simulink library "commphrec2"  (Simulink 6.0)
settings: Solver=ode45  SolverMode=SingleTasking  StartTime=0.0  StopTime=10.0  RelTol=1e-3
undefined symbols (not defined in the file or in its folder): D
libraries: commblksprivate x6, dspbuff3 x2, dspsigattribs x2, dspmathops x2, dspmtrx3 x2, simulink_extras x2
settings Model: Creator=akansal  LastModifiedBy=jli  ProdHWDeviceType=Specified
settings DataIOCC: SignalLoggingName=logsOut
settings OptimizationCC: BooleanDataType=off
settings DebuggingCC: CheckExecutionContextPreStartOutputMsg=on  CheckExecutionContextRuntimeOutputMsg=on  SolverPrmCheckMsg=none
settings HardwareCC: ProdHWDeviceType=Specified
settings ModelReferenceCC: UpdateModelReferenceTargets=IfOutOfDate
settings GRTTargetCC: LifeSpan=inf
settings SFSimCC: SFSimApplyToAllLibs=on  SFSimBuildMode=Incremental

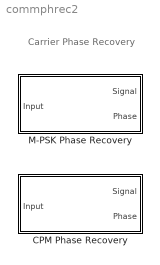
== system commphrec2 ==
  note: Carrier Phase Recovery
  CPM Phase Recovery : Subsystem  EnableExecutionContextPropagation=on  mask(CPM Phase Recovery){P=2, intPeriod=100}
      mask prompts: intPeriod "Observation interval (symbols):"
      mask help:
      | Recover the carrier phase using the 2P-Power method.  This non-data-aided, clock-aided feedforward method is suitable for full response CPM signals.
      |
      | The parameter P is the denominator of the modulation index (h=K/P) when expressed as a proper fraction. The observation interval parameter must be an integer multiple of the input signal vector length.
      mask init:
      | if ( ~isscalar(P) || (floor(P)~=P) )
      | 	error('P parameter must be an integer scalar.');
      | end
      | 
      | if ( ~isscalar(intPeriod) || (floor(intPeriod)~=intPeriod) )
      | 	error('The observation interval parameter must be an integer scalar.');
      | end
      mask Help: helpview(commbhelp);
      mask Display:
      | disp('CPM\nPhase Recovery');
      | port_label('output',1,'Sig');
      | port_label('output',2,'Ph');
  M-PSK Phase Recovery : Subsystem  EnableExecutionContextPropagation=on  mask(M-PSK Phase Recovery){M=4, intPeriod=100}
      mask prompts: M "M-ary number:"; intPeriod "Observation interval (symbols):"
      mask help:
      | Recover the carrier phase using the M-Power method.  This non-data-aided, clock-aided feedforward method is suitable for M-ary PSK modulated signals.
      |
      | The M-ary number parameter must be an even integer. The observation interval parameter must be an integer multiple of the input signal vector length.
      mask init:
      | if ( ~isscalar(M) || (mod(M,2)==1) || (floor(M)~=M) )
      | 	error('M-ary parameter must be an even integer scalar.');
      | end
      | 
      | if ( ~isscalar(intPeriod) || (floor(intPeriod)~=intPeriod) )
      | 	error('The observation interval parameter must be an integer scalar.');
      | end
      mask Help: helpview(commbhelp);
      mask Display:
      | disp('M-PSK\nPhase Recovery');
      | port_label('output',1,'Sig');
      | port_label('output',2,'Ph');

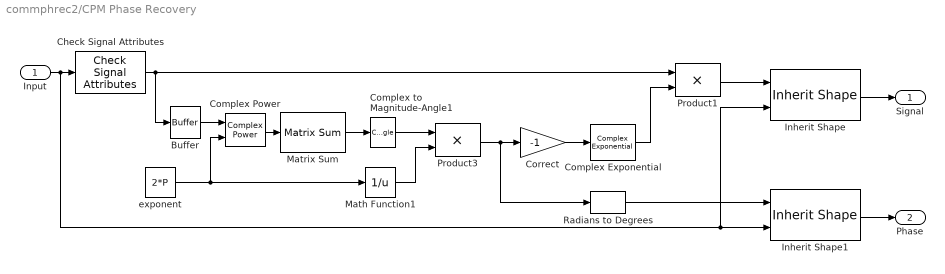
== system commphrec2/CPM Phase Recovery ==
  Input : Inport  LatchInput=off
  Buffer : dspbuff3/Buffer  N=intPeriod  V=0  ic=0
  Check Signal Attributes : dspsigattribs/Check Signal Attributes  SigAttribCheckMethod=Does not match attributes exactly  Complexity=Complex  Frame=Ignore  DimsCheckMethod=Ignore  Dimensions=1-D  DatatypeCheckMethod=Ignore  DatatypeGeneral=Boolean  DtypeFloatSpecific=Any floating-point  DtypeFixedSpecific=Any fixed-point  DtypeIntSpecific=Any integer  SampleMode=Ignore
  Complex Exponential : dspmathops/Complex Exponential
  Complex Power : commblksprivate/Complex Power
  Complex to Magnitude-Angle1 : ComplexToMagnitudeAngle  Output=Angle
  Correct : Gain  Gain=-1  SaturateOnIntegerOverflow=on
  Inherit Shape : commblksprivate/Inherit Shape
  Inherit Shape1 : commblksprivate/Inherit Shape
  Math Function1 : Math  Operator=reciprocal  SaturateOnIntegerOverflow=on
  Matrix Sum : dspmtrx3/Matrix Sum  Dim=Columns  roundingMode=Floor  overflowMode=off
  Product1 : Product  SaturateOnIntegerOverflow=on
  Product3 : Product  SaturateOnIntegerOverflow=on
  Radians to Degrees : simulink_extras/Transformations/Radians to Degrees
  exponent : Constant  Value=2*P
  Signal : Outport
  Phase : Outport  Port=2
  wires:
  Complex Exponential/1 -> Product1/2
  Matrix Sum/1 -> Complex to Magnitude-Angle1/1
  Complex to Magnitude-Angle1/1 -> Product3/1
  Input/1 -> Check Signal Attributes/1, Inherit Shape1/2, Inherit Shape/2
  Math Function1/1 -> Product3/2
  Correct/1 -> Complex Exponential/1
  Complex Power/1 -> Matrix Sum/1
  Check Signal Attributes/1 -> Product1/1, Buffer/1
  exponent/1 -> Math Function1/1, Complex Power/2
  Product3/1 -> Correct/1, Radians to Degrees/1
  Buffer/1 -> Complex Power/1
  Product1/1 -> Inherit Shape/1
  Inherit Shape/1 -> Signal/1
  Inherit Shape1/1 -> Phase/1
  Radians to Degrees/1 -> Inherit Shape1/1

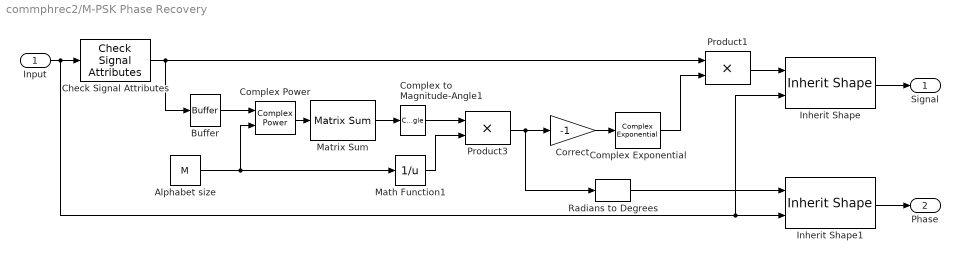
== system commphrec2/M-PSK Phase Recovery ==
  Input : Inport  LatchInput=off
  Alphabet size : Constant  Value=M
  Buffer : dspbuff3/Buffer  N=intPeriod  V=0  ic=0
  Check Signal Attributes : dspsigattribs/Check Signal Attributes  SigAttribCheckMethod=Does not match attributes exactly  Complexity=Complex  Frame=Ignore  DimsCheckMethod=Ignore  Dimensions=1-D  DatatypeCheckMethod=Ignore  DatatypeGeneral=Boolean  DtypeFloatSpecific=Any floating-point  DtypeFixedSpecific=Any fixed-point  DtypeIntSpecific=Any integer  SampleMode=Ignore
  Complex Exponential : dspmathops/Complex Exponential
  Complex Power : commblksprivate/Complex Power
  Complex to Magnitude-Angle1 : ComplexToMagnitudeAngle  Output=Angle
  Correct : Gain  Gain=-1  SaturateOnIntegerOverflow=on
  Inherit Shape : commblksprivate/Inherit Shape
  Inherit Shape1 : commblksprivate/Inherit Shape
  Math Function1 : Math  Operator=reciprocal  SaturateOnIntegerOverflow=on
  Matrix Sum : dspmtrx3/Matrix Sum  Dim=Columns  roundingMode=Floor  overflowMode=off
  Product1 : Product  SaturateOnIntegerOverflow=on
  Product3 : Product  SaturateOnIntegerOverflow=on
  Radians to Degrees : simulink_extras/Transformations/Radians to Degrees
  Signal : Outport
  Phase : Outport  Port=2
  wires:
  Alphabet size/1 -> Math Function1/1, Complex Power/2
  Check Signal Attributes/1 -> Product1/1, Buffer/1
  Complex Power/1 -> Matrix Sum/1
  Correct/1 -> Complex Exponential/1
  Math Function1/1 -> Product3/2
  Product3/1 -> Correct/1, Radians to Degrees/1
  Input/1 -> Check Signal Attributes/1, Inherit Shape1/2, Inherit Shape/2
  Complex to Magnitude-Angle1/1 -> Product3/1
  Matrix Sum/1 -> Complex to Magnitude-Angle1/1
  Complex Exponential/1 -> Product1/2
  Buffer/1 -> Complex Power/1
  Product1/1 -> Inherit Shape/1
  Inherit Shape/1 -> Signal/1
  Inherit Shape1/1 -> Phase/1
  Radians to Degrees/1 -> Inherit Shape1/1
